simulink model "model"  (R2018b)
settings: Solver=ode4  StartTime=0.0  StopTime=100  FixedStep=0.05  RelTol=1e-3
undefined symbols (not defined in the file or in its folder): degtorad
libraries: simulink x1
settings Model: Creator=Tomo  LastModifiedBy=Tomo
settings SolverCC: AlgebraicLoopSolver=LineSearch
settings DebuggingCC: AlgebraicLoopMsg=none

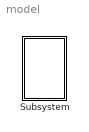
== system model ==
  Subsystem : Subsystem  mask{dt=0.003, g=9.81, k=0.7, m=2, x0=0, y0=0, v0=20, alph=45}

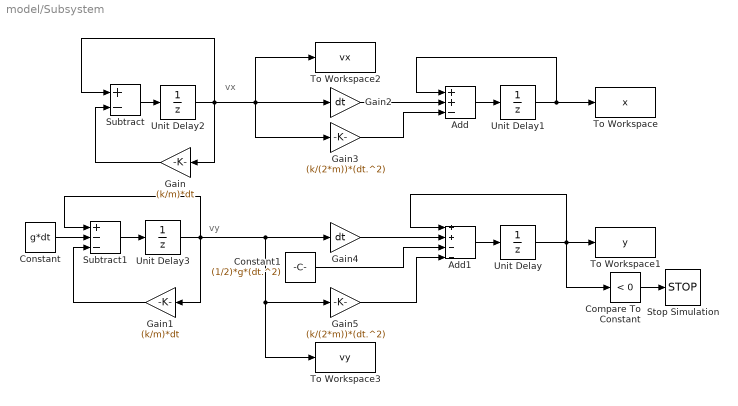
== system model/Subsystem ==
  note: vy
  note: vx
  Add : Sum  Inputs=++-
  Add1 : Sum  Inputs=++--
  Compare To Constant : simulink/Logic and Bit Operations/Compare To Constant  relop=<  const=0  OutDataTypeStr=boolean
  Constant : Constant  Value=g*dt
  Constant1 : Constant  Value=(1/2)*g*(dt.^2)
  Gain : Gain  Gain=(k/m)*dt
  Gain1 : Gain  Gain=(k/m)*dt
  Gain2 : Gain  Gain=dt
  Gain3 : Gain  Gain=(k/(2*m))*(dt.^2)
  Gain4 : Gain  Gain=dt
  Gain5 : Gain  Gain=(k/(2*m))*(dt.^2)
  Stop Simulation : Stop
  Subtract : Sum  Inputs=+-
  Subtract1 : Sum  Inputs=+--
  To Workspace : ToWorkspace  VariableName=x  SampleTime=-1
      settings: Save2DSignal=2-D array (concatenate along first dimension)
  To Workspace1 : ToWorkspace  VariableName=y  SampleTime=-1
      settings: Save2DSignal=2-D array (concatenate along first dimension)
  To Workspace2 : ToWorkspace  VariableName=vx  SampleTime=-1
      settings: Save2DSignal=2-D array (concatenate along first dimension)
  To Workspace3 : ToWorkspace  VariableName=vy  SampleTime=-1
      settings: Save2DSignal=2-D array (concatenate along first dimension)
  Unit Delay : UnitDelay  InitialCondition=y0  SampleTime=-1
  Unit Delay1 : UnitDelay  InitialCondition=x0  SampleTime=-1
  Unit Delay2 : UnitDelay  InitialCondition=v0*cos(degtorad(alph))  SampleTime=-1
  Unit Delay3 : UnitDelay  InitialCondition=v0*sin(degtorad(alph))  SampleTime=-1
  wires:
  Gain3/1 -> Add/3
  Gain5/1 -> Add1/4
  Add/1 -> Unit Delay1/1
  Subtract/1 -> Unit Delay2/1
  Constant/1 -> Subtract1/2
  Gain2/1 -> Add/2
  Constant1/1 -> Add1/3
  Gain/1 -> Subtract/2
  Gain1/1 -> Subtract1/3
  Gain4/1 -> Add1/2
  Unit Delay2/1 -> Gain/1, Gain3/1, To Workspace2/1, Gain2/1, Subtract/1
  Subtract1/1 -> Unit Delay3/1
  Unit Delay3/1 -> Gain1/1, Subtract1/1, To Workspace3/1, Gain5/1, Gain4/1
  Add1/1 -> Unit Delay/1
  Unit Delay/1 -> Compare To Constant/1, Add1/1, To Workspace1/1
  Unit Delay1/1 -> Add/1, To Workspace/1
  Compare To Constant/1 -> Stop Simulation/1
